simulink model "Base_INS"  (R2018b)
settings: configuration reference "ins_config" (kept outside this file)
undefined symbols (not defined in the file): DiscIntNeverNeededParam, INS_CONST, INS_EXPORT, INS_PARAM
libraries: simulink x95, AP_Math x15, Filter x6, Quaternion x2, Rotation x2
(part 1 of 4)
settings Model: SimulationMode=accelerator  Creator=Jiachi  LastModifiedBy=zouji
settings ConfigSetRef: SourceLocation=Base Workspace

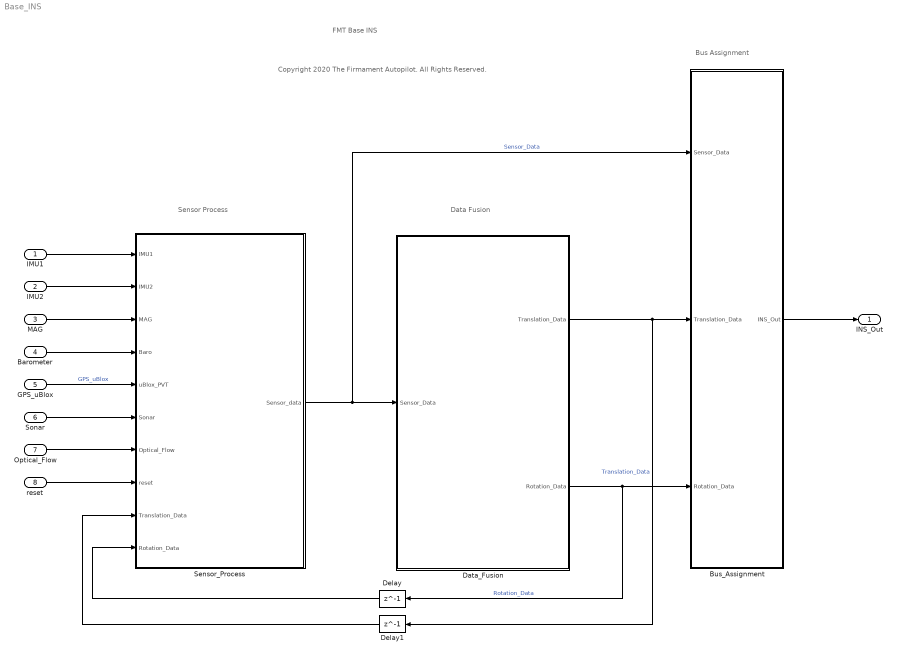
== system Base_INS ==
  note: FMT Base INS
  note: Sensor Process
  note: Data Fusion
  note: Bus Assignment
  note: Copyright 2020 The Firmament Autopilot. All Rights Reserved.
  IMU1 : Inport  OutDataTypeStr=Bus: IMU_Bus  PortDimensions=[1 1]  SampleTime=[INS_CONST.dt,0]  Interpolate=off  BusOutputAsStruct=on
  IMU2 : Inport  Port=2  OutDataTypeStr=Bus: IMU_Bus  PortDimensions=[1 1]  SampleTime=[INS_CONST.dt,0]  Interpolate=off  BusOutputAsStruct=on
  MAG : Inport  Port=3  OutDataTypeStr=Bus: MAG_Bus  PortDimensions=[1 1]  SampleTime=[INS_CONST.dt,0]  Interpolate=off  BusOutputAsStruct=on
  Barometer : Inport  Port=4  OutDataTypeStr=Bus: Barometer_Bus  PortDimensions=[1 1]  SampleTime=[INS_CONST.dt,0]  Interpolate=off  BusOutputAsStruct=on
  GPS_uBlox : Inport  Port=5  OutDataTypeStr=Bus: GPS_uBlox_Bus  PortDimensions=[1 1]  SampleTime=[INS_CONST.dt,0]  Interpolate=off  BusOutputAsStruct=on
  Sonar : Inport  Port=6  OutDataTypeStr=Bus: Sonar_Bus  PortDimensions=1  SampleTime=[INS_CONST.dt,0]  Interpolate=off  BusOutputAsStruct=on
  Optical_Flow : Inport  Port=7  OutDataTypeStr=Bus: Optical_Flow_Bus  PortDimensions=[1 1]  SampleTime=[INS_CONST.dt,0]  Interpolate=off  BusOutputAsStruct=on
  reset : Inport  Port=8  OutDataTypeStr=uint8  PortDimensions=1
  Bus_Assignment : Subsystem  TreatAsAtomicUnit=on
  Data_Fusion : Subsystem  TreatAsAtomicUnit=on
  Delay : Delay  DelayLength=1
  Delay1 : Delay  DelayLength=1
  Sensor_Process : Subsystem  TreatAsAtomicUnit=on
  INS_Out : Outport  OutDataTypeStr=Bus: INS_Out_Bus
  wires:
  IMU1/1 -> Sensor_Process/1(IMU1)
  MAG/1 -> Sensor_Process/3(MAG)
  Barometer/1 -> Sensor_Process/4(Baro)
  GPS_uBlox/1 -> Sensor_Process/5(uBlox_PVT)  "GPS_uBlox"
  Sonar/1 -> Sensor_Process/6(Sonar)
  Bus_Assignment/1(INS_Out) -> INS_Out/1
  reset/1 -> Sensor_Process/8(reset)
  Optical_Flow/1 -> Sensor_Process/7(Optical_Flow)
  IMU2/1 -> Sensor_Process/2(IMU2)
  Sensor_Process/1(Sensor_data) -> Bus_Assignment/1(Sensor_Data), Data_Fusion/1(Sensor_Data)  "Sensor_Data"
  Data_Fusion/2(Rotation_Data) -> Delay/1, Bus_Assignment/3(Rotation_Data)  "Rotation_Data"
  Data_Fusion/1(Translation_Data) -> Delay1/1, Bus_Assignment/2(Translation_Data)  "Translation_Data"
  Delay/1 -> Sensor_Process/10(Rotation_Data)
  Delay1/1 -> Sensor_Process/9(Translation_Data)

== system Base_INS/Bus_Assignment ==
  Sensor_Data : Inport
  Translation_Data : Inport  Port=2
  Rotation_Data : Inport  Port=3
  Bus Creator : BusCreator  Inputs=24  OutDataTypeStr=Bus: INS_Out_Bus
      settings: InheritFromInputs=off
  Counter : Subsystem  TreatAsAtomicUnit=on
  Rotation_Output : Subsystem  TreatAsAtomicUnit=on
  Status_Output : Subsystem  TreatAsAtomicUnit=on
  Translation_Output : Subsystem  TreatAsAtomicUnit=on
  INS_Out : Outport  OutDataTypeStr=Bus: INS_Out_Bus
  wires:
  Bus Creator/1 -> INS_Out/1
  Counter/1(timestamp_ms) -> Bus Creator/1  "timestamp"
  Rotation_Output/2(theta) -> Bus Creator/3  "theta"
  Rotation_Output/1(phi) -> Bus Creator/2  "phi"
  Rotation_Output/4(att_quat) -> Bus Creator/5  "quat"
  Rotation_Output/3(psi) -> Bus Creator/4  "psi"
  Rotation_Output/5(p) -> Bus Creator/6  "p"
  Rotation_Output/6(q) -> Bus Creator/7  "q"
  Rotation_Output/7(r) -> Bus Creator/8  "r"
  Rotation_Output/8(sfor_x) -> Bus Creator/9  "ax"
  Rotation_Output/9(sfor_y) -> Bus Creator/10  "ay"
  Rotation_Output/10(sfor_z) -> Bus Creator/11  "az"
  Translation_Output/1(velN) -> Bus Creator/12  "vn"
  Translation_Output/2(velE) -> Bus Creator/13  "ve"
  Translation_Output/3(velD) -> Bus Creator/14  "vd"
  Translation_Output/5(longitude) -> Bus Creator/16  "lon"
  Translation_Output/6(latitude) -> Bus Creator/17  "lat"
  Translation_Output/7(altitude) -> Bus Creator/18  "alt"
  Status_Output/1(flag) -> Bus Creator/23  "flag"
  Status_Output/2(status) -> Bus Creator/24  "status"
  Translation_Output/8(x_R_m) -> Bus Creator/19  "x_R"
  Translation_Output/9(y_R_m) -> Bus Creator/20  "y_R"
  Translation_Output/10(h_R_m) -> Bus Creator/21  "h_R"
  Translation_Output/11(h_AGL_m) -> Bus Creator/22  "h_AGL"
  Translation_Output/4(reserved) -> Bus Creator/15  "reserved"
  Translation_Data/1 -> Status_Output/1(Translation_Data), Translation_Output/1(Translation_Data), Rotation_Output/2(Translation_Data)
  Rotation_Data/1 -> Status_Output/2(Rotation_Data), Rotation_Output/1(Rotation_Data)
  Sensor_Data/1 -> Status_Output/3(Sensor_Data)

== system Base_INS/Data_Fusion ==
  note: AHRS
  note: Translaton Filter
  Sensor_Data : Inport
  AHRS : Subsystem
  Translation_Filter : Subsystem
  Translation_Data : Outport
  Rotation_Data : Outport  Port=2
  wires:
  AHRS/1(Rotation_Data) -> Rotation_Data/1, Translation_Filter/2(Rotation_Data)
  Translation_Filter/1(Translation_Data) -> Translation_Data/1
  Sensor_Data/1 -> Translation_Filter/1(Sensor_Data), AHRS/1(Sensor_Data)

== system Base_INS/Sensor_Process ==
  IMU1 : Inport  Interpolate=off  BusOutputAsStruct=on
  IMU2 : Inport  Port=2  Interpolate=off  BusOutputAsStruct=on
  MAG : Inport  Port=3  Interpolate=off  BusOutputAsStruct=on
  Baro : Inport  Port=4  Interpolate=off  BusOutputAsStruct=on
  uBlox_PVT : Inport  Port=5  Interpolate=off  BusOutputAsStruct=on
  Sonar : Inport  Port=6  PortDimensions=[1 1]  Interpolate=off  BusOutputAsStruct=on
  Optical_Flow : Inport  Port=7
  reset : Inport  Port=8
  Translation_Data : Inport  Port=9
  Rotation_Data : Inport  Port=10
  Baro_Process : Subsystem  TreatAsAtomicUnit=on
  Bus Creator : BusCreator  Inputs=7
  GPS_Process : Subsystem  TreatAsAtomicUnit=on
  IMU_Process : Subsystem  TreatAsAtomicUnit=on
  Mag_Process : Subsystem  TreatAsAtomicUnit=on
  Optical_Flow_Preprocessing : Subsystem  TreatAsAtomicUnit=on
  Signal Conversion : SignalConversion  OverrideOpt=off
  Sonar_Process : Subsystem  TreatAsAtomicUnit=on
  Sensor_data : Outport
  wires:
  Translation_Data/1 -> Sonar_Process/1(Translation_Data)
  Sonar_Process/1(Sonar_Data) -> Bus Creator/5  "Sonar_Data"
  Sonar/1 -> Sonar_Process/2(Sonar)
  IMU1/1 -> IMU_Process/1(IMU1)
  uBlox_PVT/1 -> GPS_Process/1(uBlox_PVT)
  GPS_Process/1(GPS_Data) -> Mag_Process/3(GPS_Data), Bus Creator/3  "GPS_Data"
  MAG/1 -> Mag_Process/1(Mag)
  Rotation_Data/1 -> Optical_Flow_Preprocessing/1(Rotation_Data), Mag_Process/2(Rotation_Data)
  Baro/1 -> Baro_Process/1(Baro)
  IMU_Process/1(IMU_Data) -> Bus Creator/1  "IMU_Data"
  Mag_Process/1(Mag_Data) -> Bus Creator/2  "Mag_Data"
  reset/1 -> Signal Conversion/1
  Signal Conversion/1 -> Bus Creator/7  "global_reset"
  Baro_Process/1(Baro_Data) -> Bus Creator/4  "Baro_Data"
  Bus Creator/1 -> Sensor_data/1
  Optical_Flow/1 -> Optical_Flow_Preprocessing/2(Vision_Flow)
  Optical_Flow_Preprocessing/1(VisionFlow_Data) -> Bus Creator/6  "VisionFlow_Data"
  IMU2/1 -> IMU_Process/2(IMU2)

== system Base_INS/Bus_Assignment/Counter ==
  Add : Sum
  Constant : Constant  Value=INS_EXPORT.period  OutDataTypeStr=uint32
  Data Type Conversion : DataTypeConversion  OutDataTypeStr=uint32
  Output : UnitDelay  InitialCondition=0.0  SampleTime=-1
  timestamp_ms : Outport
  wires:
  Add/1 -> Output/1
  Output/1 -> Add/2, Data Type Conversion/1
  Data Type Conversion/1 -> timestamp_ms/1
  Constant/1 -> Add/1

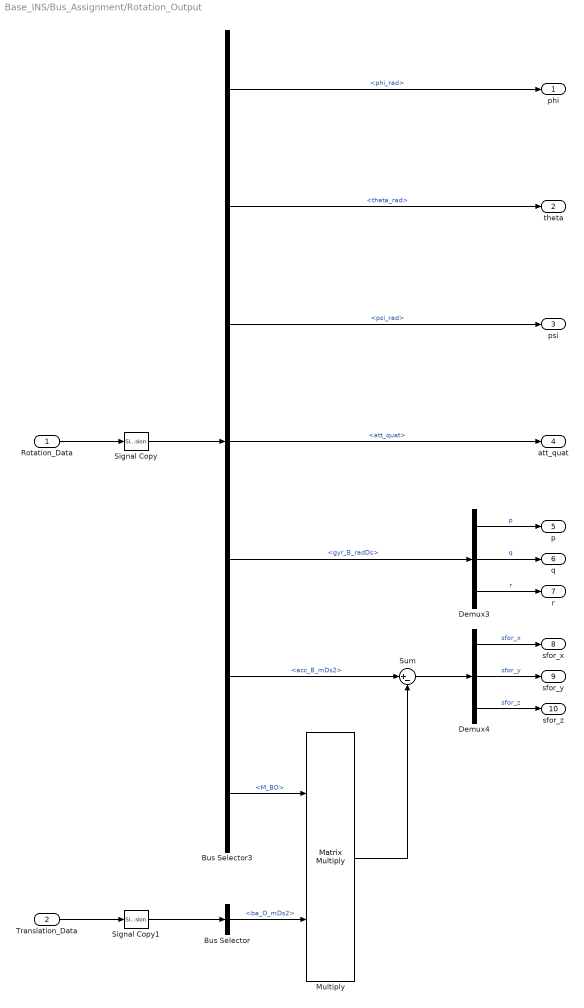
== system Base_INS/Bus_Assignment/Rotation_Output ==
  Rotation_Data : Inport
  Translation_Data : Inport  Port=2
  Bus Selector : BusSelector  OutputSignals=ba_O_mDs2
  Bus Selector3 : BusSelector  OutputSignals=phi_rad,theta_rad,psi_rad,att_quat,gyr_B_radDs,acc_B_mDs2,M_BO
  Demux3 : Demux  Outputs=3
  Demux4 : Demux  Outputs=3
  Multiply : Product  Multiplication=Matrix(*)
  Signal Copy : SignalConversion  OverrideOpt=off
  Signal Copy1 : SignalConversion  OverrideOpt=off
  Sum : Sum  Inputs=|+-
  phi : Outport
  theta : Outport  Port=2
  psi : Outport  Port=3
  att_quat : Outport  Port=4
  p : Outport  Port=5
  q : Outport  Port=6
  r : Outport  Port=7
  sfor_x : Outport  Port=8
  sfor_y : Outport  Port=9
  sfor_z : Outport  Port=10
  wires:
  Bus Selector/1 -> Multiply/2  "<ba_O_mDs2>"
  Demux4/1 -> sfor_x/1  "sfor_x"
  Demux3/3 -> r/1  "r"
  Demux3/2 -> q/1  "q"
  Demux3/1 -> p/1  "p"
  Bus Selector3/5 -> Demux3/1  "<gyr_B_radDs>"
  Sum/1 -> Demux4/1
  Bus Selector3/1 -> phi/1  "<phi_rad>"
  Bus Selector3/6 -> Sum/1  "<acc_B_mDs2>"
  Demux4/3 -> sfor_z/1  "sfor_z"
  Demux4/2 -> sfor_y/1  "sfor_y"
  Bus Selector3/2 -> theta/1  "<theta_rad>"
  Bus Selector3/3 -> psi/1  "<psi_rad>"
  Bus Selector3/7 -> Multiply/1  "<M_BO>"
  Multiply/1 -> Sum/2
  Bus Selector3/4 -> att_quat/1  "<att_quat>"
  Rotation_Data/1 -> Signal Copy/1
  Translation_Data/1 -> Signal Copy1/1
  Signal Copy/1 -> Bus Selector3/1
  Signal Copy1/1 -> Bus Selector/1

== system Base_INS/Bus_Assignment/Status_Output ==
  Translation_Data : Inport
  Rotation_Data : Inport  Port=2
  Sensor_Data : Inport  Port=3
  Bus Selector2 : BusSelector  OutputSignals=standstill
  INS_Flag : Subsystem
  INS_Quality : Subsystem
  INS_Ready : Subsystem
  Sensor_Status : Subsystem
  flag : Outport
  status : Outport  Port=2
  wires:
  INS_Flag/1(flags) -> flag/1
  Sensor_Status/1(status) -> status/1
  INS_Quality/1(Quality) -> INS_Flag/2(INS_Quality)
  Rotation_Data/1 -> INS_Ready/2(Rotation_Data), Bus Selector2/1
  Sensor_Data/1 -> INS_Quality/1(Sensor_Data), INS_Flag/3(Sensor_Data), Sensor_Status/1(Sensor_Data)
  Bus Selector2/1 -> INS_Flag/4(standstill)  "<standstill>"
  Translation_Data/1 -> INS_Ready/1(Translation_Data)
  INS_Ready/1(INS_Ready) -> INS_Flag/1(INS_ready)

== system Base_INS/Bus_Assignment/Translation_Output ==
  Translation_Data : Inport
  Bus Selector4 : BusSelector  OutputSignals=vel_N_mDs,vel_E_mDs,vel_D_mDs,mue_rad,lambda_rad,h_m,x_R_m,y_R_m,h_R_m,h_gnd_m
  Constant : Constant  Value=0  OutDataTypeStr=single
  Signal Copy : SignalConversion  OverrideOpt=off
  velN : Outport
  velE : Outport  Port=2
  velD : Outport  Port=3
  reserved : Outport  Port=4
  longitude : Outport  Port=5
  latitude : Outport  Port=6
  altitude : Outport  Port=7
  x_R_m : Outport  Port=8
  y_R_m : Outport  Port=9
  h_R_m : Outport  Port=10
  h_AGL_m : Outport  Port=11
  wires:
  Translation_Data/1 -> Signal Copy/1
  Bus Selector4/4 -> latitude/1  "<mue_rad>"
  Bus Selector4/5 -> longitude/1  "<lambda_rad>"
  Bus Selector4/2 -> velE/1  "<vel_E_mDs>"
  Bus Selector4/3 -> velD/1  "<vel_D_mDs>"
  Bus Selector4/6 -> altitude/1  "<h_m>"
  Bus Selector4/1 -> velN/1  "<vel_N_mDs>"
  Bus Selector4/10 -> h_AGL_m/1  "<h_gnd_m>"
  Bus Selector4/9 -> h_R_m/1  "<h_R_m>"
  Bus Selector4/7 -> x_R_m/1  "<x_R_m>"
  Bus Selector4/8 -> y_R_m/1  "<y_R_m>"
  Constant/1 -> reserved/1
  Signal Copy/1 -> Bus Selector4/1

== system Base_INS/Data_Fusion/AHRS ==
  Sensor_Data : Inport
  Attitude_Init : Subsystem  TreatAsAtomicUnit=on
  Correct : Subsystem  TreatAsAtomicUnit=on
  Delay : Delay  DelayLength=1
  Integrate : Subsystem  TreatAsAtomicUnit=on
  Rotation_Data : Outport
  wires:
  Correct/1(rot_B_correction) -> Integrate/1(rot_B_correction)
  Correct/2(bias_g_correction) -> Integrate/2(bias_g_correction)
  Attitude_Init/1(standstill) -> Integrate/3(standstill), Correct/3(standstill)
  Integrate/1(Rotation_Data) -> Rotation_Data/1, Delay/1
  Attitude_Init/3(quat_0) -> Integrate/5(quat_0)
  Attitude_Init/2(att_reset) -> Integrate/4(att_reset)
  Sensor_Data/1 -> Integrate/6(Sensor_Data), Correct/2(Sensor_Data), Attitude_Init/1(Sensor_Data)
  Delay/1 -> Correct/1(Rotation_Data)

== system Base_INS/Data_Fusion/Translation_Filter ==
  Sensor_Data : Inport
  Rotation_Data : Inport  Port=2
  CF : Subsystem  TreatAsAtomicUnit=on
  Delay : Delay  DelayLength=1
  Process : Subsystem  TreatAsAtomicUnit=on
  Translation_Data : Outport
  wires:
  CF/1(Translation_Data) -> Delay/1, Translation_Data/1
  Process/1(Processed_Data) -> CF/1(Processed_Data)  "Processed_Data"
  Rotation_Data/1 -> CF/2(Rotation_Data), Process/2(Rotation_Data)
  Sensor_Data/1 -> Process/1(Sensor_Data)
  Delay/1 -> Process/3(Translation_Data)

== system Base_INS/Sensor_Process/Baro_Process ==
  Baro : Inport
  Bus Creator : BusCreator  Inputs=5
  Bus Selector1 : BusSelector  OutputSignals=pressure
  Bus Selector2 : BusSelector  OutputSignals=temperature,timestamp
  P1 : Constant  Value=101.325  OutDataTypeStr=Inherit: Inherit via back propagation
  Pressure_Height : Subsystem
  Relative_Height : Subsystem  mask{pressure_min=30e3, pressure_max=110e3, temp_min=-30, temp_max=80, s_first=500, s_last=1000}
      mask prompts: pressure_min "Min. valid pressure"; pressure_max "Max. valid pressure"; temp_min "Min. valid temperature"; temp_max "Max. valid temperature"; s_first "First Sample for Initial Averaging"; s_last "Last Sample for Initial Averaging"
  Baro_Data : Outport
  wires:
  Bus Selector1/1 -> Pressure_Height/1(p_Pa)  "<pressure>"
  P1/1 -> Pressure_Height/2(QNH_kPa)
  Relative_Height/2(valid) -> Bus Creator/2  "baro_valid"
  Baro/1 -> Bus Selector2/1, Bus Selector1/1, Relative_Height/1(Baro)
  Relative_Height/1(h_R_m) -> Bus Creator/1  "h_R_m"
  Pressure_Height/1(h_FL_m) -> Bus Creator/3  "h_FL_m"
  Bus Creator/1 -> Baro_Data/1
  Bus Selector2/1 -> Bus Creator/4  "<temperature>"
  Bus Selector2/2 -> Bus Creator/5  "<timestamp>"

== system Base_INS/Sensor_Process/GPS_Process ==
  uBlox_PVT : Inport  Interpolate=off  BusOutputAsStruct=on
  Bus Creator1 : BusCreator  Inputs=16
  Compare To Constant : simulink/Logic and Bit Operations/Compare To Constant  relop=>  const=0  OutDataTypeStr=boolean
  Compare To Constant1 : simulink/Logic and Bit Operations/Compare To Constant  relop=<  const=2  OutDataTypeStr=boolean
  GPS_Status_and_Quality : Subsystem
  Scaling : Subsystem
  WGS84_Model : Subsystem
  GPS_Data : Outport
  wires:
  Compare To Constant1/1 -> Bus Creator1/1  "GPS_reset"
  WGS84_Model/5(dz_dh) -> Bus Creator1/8  "dz_dh"
  uBlox_PVT/1 -> Scaling/1(uBlox_PVT), GPS_Status_and_Quality/1(uBlox_PVT)
  Compare To Constant/1 -> WGS84_Model/Trigger
  Bus Creator1/1 -> GPS_Data/1
  GPS_Status_and_Quality/1(gps_status) -> Compare To Constant1/1, Compare To Constant/1  "Status"
  WGS84_Model/2(lat_0_rad) -> Bus Creator1/5  "lat_0_rad"
  WGS84_Model/3(dx_dlat) -> Bus Creator1/6
  WGS84_Model/4(dy_dlon) -> Bus Creator1/7
  GPS_Status_and_Quality/2(speed_quality) -> Bus Creator1/2  "sqd_quality"
  GPS_Status_and_Quality/3(pos_quality) -> Bus Creator1/3  "pos_quality"
  Scaling/2(lon_rad) -> WGS84_Model/2(lon), Bus Creator1/10  "lambda_rad"
  Scaling/3(height_m) -> WGS84_Model/3(height), Bus Creator1/11  "height_m"
  Scaling/1(lat_rad) -> Bus Creator1/9, WGS84_Model/1(lat)  "mue_rad"
  Scaling/4(vel_N) -> Bus Creator1/12  "vn_mPs"
  Scaling/5(vel_E) -> Bus Creator1/13  "ve_mPs"
  Scaling/6(vel_D) -> Bus Creator1/14  "vd_mPs"
  Scaling/7(numSV) -> Bus Creator1/15  "numSV"
  Scaling/8(timestamp_ms) -> Bus Creator1/16  "timestamp_ms"
  WGS84_Model/1(lon_0_rad) -> Bus Creator1/4  "lon_0_rad"

== system Base_INS/Sensor_Process/IMU_Process ==
  IMU1 : Inport
  IMU2 : Inport  Port=2
  Bus Creator : BusCreator  Inputs=4
  Bus_Assignment : Subsystem
  IMU1_Scaling : Subsystem
  IMU1_Valid_Check : Subsystem  mask{gyr_min=-2200*pi/180, gyr_max=2200*pi/180, acc_min=-10*INS_CONST.g, acc_max=10*INS_CONST.g, timeout=100}
      mask prompts: gyr_min "Gyro Min Value"; gyr_max "Gyro Max Value"; acc_min "Accel Min Value"; acc_max "Accel Max Value"; timeout "Timeout in ms"
  IMU2_Scaling : Subsystem
  IMU2_Valid_Check : Subsystem  mask{gyr_min=-2200*pi/180, gyr_max=2200*pi/180, acc_min=-10*INS_CONST.g, acc_max=10*INS_CONST.g, timeout=100}
      mask prompts: gyr_min "Gyro Min Value"; gyr_max "Gyro Max Value"; acc_min "Accel Min Value"; acc_max "Accel Max Value"; timeout "Timeout in ms"
  IMU_Data : Outport
  wires:
  Bus Creator/1 -> IMU_Data/1
  IMU2_Scaling/3(timestamp_ms) -> IMU2_Valid_Check/3(timestamp_ms)
  IMU2_Scaling/2(acc_B_mDs2) -> IMU2_Valid_Check/2(acc_B_mDs2), Bus_Assignment/5(IMU2_acc_B_mPs2)
  IMU2_Scaling/1(gyr_B_radDs) -> IMU2_Valid_Check/1(gyr_B_radDs), Bus_Assignment/4(IMU2_gyr_B_radPs)
  IMU2/1 -> IMU2_Scaling/1(IMU2)
  IMU1_Scaling/1(gyr_B_radDs) -> IMU1_Valid_Check/1(gyr_B_radDs), Bus_Assignment/1(IMU1_gyr_B_radPs)
  IMU1/1 -> IMU1_Scaling/1(IMU1)
  IMU1_Scaling/3(timestamp_ms) -> IMU1_Valid_Check/3(timestamp_ms)
  IMU1_Scaling/2(acc_B_mDs2) -> IMU1_Valid_Check/2(acc_B_mDs2), Bus_Assignment/2(IMU1_acc_B_mPs2)
  IMU1_Valid_Check/1(valid) -> Bus_Assignment/3(IMU1_valid)  "IMU1_valid"
  IMU2_Valid_Check/1(valid) -> Bus_Assignment/6(IMU2_valid)  "IMU2_valid"
  Bus_Assignment/1(gyr_B_radPs) -> Bus Creator/1  "gyr_B_radPs"
  Bus_Assignment/2(acc_B_mPs2) -> Bus Creator/2  "acc_B_mPs2"
  Bus_Assignment/3(IMU_status) -> Bus Creator/3  "IMU_status"
  Bus_Assignment/4(IMU_valid) -> Bus Creator/4  "IMU_valid"

== system Base_INS/Sensor_Process/Mag_Process ==
  Mag : Inport
  Rotation_Data : Inport  Port=2
  GPS_Data : Inport  Port=3
  Bus Creator : BusCreator  Inputs=2
  Bus Selector : BusSelector  OutputSignals=timestamp
  Bus Selector2 : BusSelector  OutputSignals=mag_x,mag_y,mag_z
  Bus Selector4 : BusSelector  OutputSignals=M_OB
  Mag_Scaling : Subsystem
  Mag_Valid_Check : Subsystem  mask{mag_min=-30000, mag_max=30000, timeout=1000}
      mask prompts: mag_min "Min Mag Value"; mag_max "Max Mag Value"; timeout "Timeout in ms"
  Magnetometer : Subsystem
  Vector Concatenate2 : Concatenate  NumInputs=3  Mode=Multidimensional array
  Mag_Data : Outport
  wires:
  Rotation_Data/1 -> Bus Selector4/1
  Vector Concatenate2/1 -> Mag_Valid_Check/1(mag_B_gauss), Mag_Scaling/1(mag_B_gauss)
  Bus Selector2/2 -> Vector Concatenate2/2  "<mag_y>"
  Bus Selector2/1 -> Vector Concatenate2/1  "<mag_x>"
  Bus Selector4/1 -> Magnetometer/3(M_OB)  "<M_OB>"
  Mag_Valid_Check/1(valid) -> Magnetometer/2(Mag_valid)
  Bus Selector2/3 -> Vector Concatenate2/3  "<mag_z>"
  Mag_Scaling/1(mag_B_uT) -> Magnetometer/1(mag_B_uT)
  Mag/1 -> Bus Selector/1, Bus Selector2/1
  Magnetometer/1(mag_normalized_B) -> Bus Creator/1  "mag_norm_B"
  GPS_Data/1 -> Magnetometer/4(GPS_Data)
  Magnetometer/2(mag_Quality) -> Bus Creator/2  "mag_quality"
  Bus Creator/1 -> Mag_Data/1
  Bus Selector/1 -> Mag_Valid_Check/2(timestamp_ms)  "<timestamp>"

== system Base_INS/Sensor_Process/Optical_Flow_Preprocessing ==
  Rotation_Data : Inport
  Vision_Flow : Inport  Port=2
  Bus Creator : BusCreator  Inputs=6
  Bus Selector : BusSelector  OutputSignals=timestamp_ms,valid,vel_x_mPs,vel_y_mPs
  Bus Selector1 : BusSelector  OutputSignals=M_CO
  Constant : Constant  Value=0  OutDataTypeStr=single
  Demux : Demux  Outputs=3
  Multiply : Product  Multiplication=Matrix(*)
  Mux : Mux  Inputs=3
  Signal Copy{,1..3} (4 alike) : SignalConversion  OverrideOpt=off
  Terminator : Terminator
  Valid_Detect : Subsystem
  VisionFlow_Data : Outport
  wires:
  Bus Creator/1 -> VisionFlow_Data/1
  Vision_Flow/1 -> Bus Selector/1
  Bus Selector/3 -> Signal Copy/1, Mux/1  "<vel_x_mPs>"
  Bus Selector/4 -> Signal Copy1/1, Mux/2  "<vel_y_mPs>"
  Signal Copy/1 -> Bus Creator/3  "vel_x_B_mDs"
  Signal Copy1/1 -> Bus Creator/4  "vel_y_B_mDs"
  Bus Selector/1 -> Bus Creator/1, Valid_Detect/1(timestamp_ms)  "<timestamp_ms>"
  Bus Selector/2 -> Valid_Detect/2(vf_valid)  "<valid>"
  Valid_Detect/1(valid) -> Bus Creator/2  "valid"
  Rotation_Data/1 -> Bus Selector1/1
  Signal Copy2/1 -> Bus Creator/5  "vel_x_O_mDs"
  Signal Copy3/1 -> Bus Creator/6  "vel_y_O_mDs"
  Bus Selector1/1 -> Multiply/1  "<M_CO>"
  Constant/1 -> Mux/3
  Mux/1 -> Multiply/2
  Multiply/1 -> Demux/1
  Demux/1 -> Signal Copy2/1
  Demux/2 -> Signal Copy3/1
  Demux/3 -> Terminator/1

== system Base_INS/Sensor_Process/Sonar_Process ==
  Translation_Data : Inport
  Sonar : Inport  Port=2
  Bus Creator : BusCreator  Inputs=3
  Bus Selector : BusSelector  OutputSignals=timestamp_ms,distance_m
  Signal Conversion : SignalConversion  OverrideOpt=off
  Signal Conversion1 : SignalConversion  OverrideOpt=off
  Valid_Check : Subsystem
  Sonar_Data : Outport
  wires:
  Translation_Data/1 -> Valid_Check/3(Translation_Data)
  Bus Creator/1 -> Sonar_Data/1
  Signal Conversion/1 -> Bus Creator/2  "distance_m"
  Sonar/1 -> Bus Selector/1
  Bus Selector/2 -> Valid_Check/2(diatance_m), Signal Conversion/1  "<distance_m>"
  Bus Selector/1 -> Signal Conversion1/1, Valid_Check/1(timestamp_ms)  "<timestamp_ms>"
  Valid_Check/1(sonar_valid) -> Bus Creator/3  "sonar_valid"
  Signal Conversion1/1 -> Bus Creator/1  "timestamp_ms"

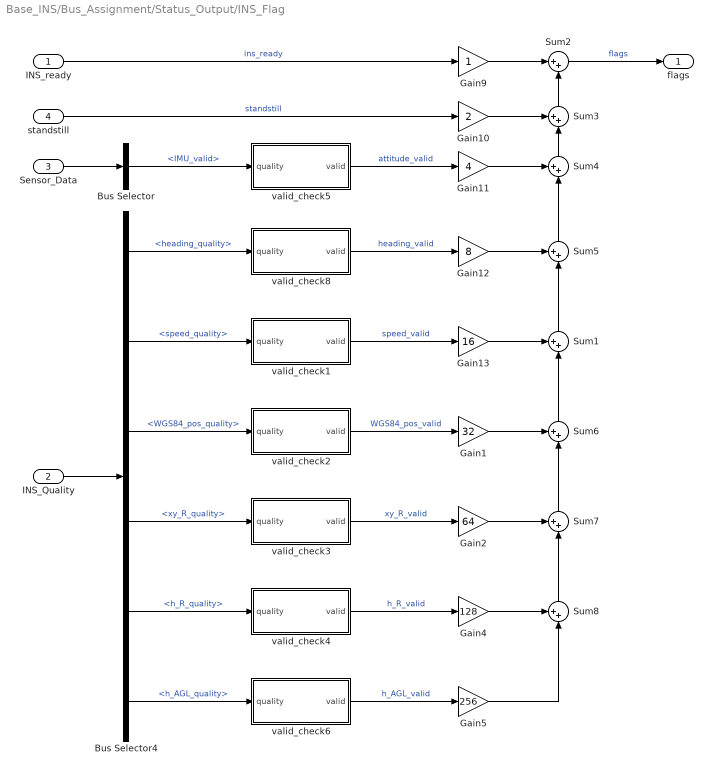
== system Base_INS/Bus_Assignment/Status_Output/INS_Flag ==
  INS_ready : Inport
  INS_Quality : Inport  Port=2
  Sensor_Data : Inport  Port=3
  standstill : Inport  Port=4
  Bus Selector : BusSelector  OutputSignals=IMU_Data.IMU_valid
  Bus Selector4 : BusSelector  OutputSignals=heading_quality,speed_quality,WGS84_pos_quality,xy_R_quality,h_R_quality,h_AGL_quality
  Gain1 : Gain  Gain=32  OutDataTypeStr=uint32
  Gain10 : Gain  Gain=2  OutDataTypeStr=uint32
  Gain11 : Gain  Gain=4  OutDataTypeStr=uint32
  Gain12 : Gain  Gain=8  OutDataTypeStr=uint32
  Gain13 : Gain  Gain=16  OutDataTypeStr=uint32
  Gain2 : Gain  Gain=64  OutDataTypeStr=uint32
  Gain4 : Gain  Gain=128  OutDataTypeStr=uint32
  Gain5 : Gain  Gain=256  OutDataTypeStr=uint32
  Gain9 : Gain  OutDataTypeStr=uint32
  Sum{1,3..8} (7 alike) : Sum  Inputs=++|
  Sum2 : Sum  Inputs=|++
  valid_check1 : Subsystem  mask{time_out=1000}
      mask prompts: time_out "timeout in ms"
  valid_check2 : Subsystem  mask{time_out=1000}
      mask prompts: time_out "timeout in ms"
  valid_check3 : Subsystem  mask{time_out=1000}
      mask prompts: time_out "timeout in ms"
  valid_check4 : Subsystem  mask{time_out=200}
      mask prompts: time_out "timeout in ms"
  valid_check5 : Subsystem  mask{time_out=100}
      mask prompts: time_out "timeout in ms"
  valid_check6 : Subsystem  mask{time_out=100}
      mask prompts: time_out "timeout in ms"
  valid_check8 : Subsystem  mask{time_out=1000}
      mask prompts: time_out "timeout in ms"
  flags : Outport
  wires:
  INS_ready/1 -> Gain9/1  "ins_ready"
  Bus Selector/1 -> valid_check5/1(quality)  "<IMU_valid>"
  Gain1/1 -> Sum6/1
  Sum1/1 -> Sum5/2
  Gain13/1 -> Sum1/1
  valid_check2/1(valid) -> Gain1/1  "WGS84_pos_valid"
  valid_check1/1(valid) -> Gain13/1  "speed_valid"
  valid_check5/1(valid) -> Gain11/1  "attitude_valid"
  Bus Selector4/3 -> valid_check2/1(quality)  "<WGS84_pos_quality>"
  Bus Selector4/2 -> valid_check1/1(quality)  "<speed_quality>"
  Bus Selector4/1 -> valid_check8/1(quality)  "<heading_quality>"
  INS_Quality/1 -> Bus Selector4/1
  Sum2/1 -> flags/1  "flags"
  Sum5/1 -> Sum4/2
  Gain9/1 -> Sum2/1
  Gain11/1 -> Sum4/1
  Gain12/1 -> Sum5/1
  Sum3/1 -> Sum2/2
  Sum4/1 -> Sum3/2
  Sensor_Data/1 -> Bus Selector/1
  Gain10/1 -> Sum3/1
  Sum6/1 -> Sum1/2
  Sum7/1 -> Sum6/2
  standstill/1 -> Gain10/1  "standstill"
  valid_check3/1(valid) -> Gain2/1  "xy_R_valid"
  valid_check4/1(valid) -> Gain4/1  "h_R_valid"
  Gain2/1 -> Sum7/1
  Sum8/1 -> Sum7/2
  Gain4/1 -> Sum8/1
  Gain5/1 -> Sum8/2
  valid_check6/1(valid) -> Gain5/1  "h_AGL_valid"
  Bus Selector4/4 -> valid_check3/1(quality)  "<xy_R_quality>"
  Bus Selector4/5 -> valid_check4/1(quality)  "<h_R_quality>"
  Bus Selector4/6 -> valid_check6/1(quality)  "<h_AGL_quality>"
  valid_check8/1(valid) -> Gain12/1  "heading_valid"

== system Base_INS/Bus_Assignment/Status_Output/INS_Quality ==
  Sensor_Data : Inport
  Bus Creator : BusCreator  Inputs=6
  Bus Selector : BusSelector  OutputSignals=GPS_Data.sqd_quality
  Bus Selector1 : BusSelector  OutputSignals=GPS_Data.pos_quality
  Bus Selector2 : BusSelector  OutputSignals=Mag_Data.mag_quality
  Bus Selector3 : BusSelector  OutputSignals=GPS_Data.sqd_quality
  Bus Selector4 : BusSelector  OutputSignals=VisionFlow_Data.valid
  Bus Selector5 : BusSelector  OutputSignals=Baro_Data.baro_valid
  Bus Selector6 : BusSelector  OutputSignals=Sonar_Data.sonar_valid
  Data Type Conversion : DataTypeConversion  OutDataTypeStr=single
  Data Type Conversion1 : DataTypeConversion  OutDataTypeStr=single
  Data Type Conversion2 : DataTypeConversion  OutDataTypeStr=single
  Max : MinMax  Function=max  Inputs=2
  Max1 : MinMax  Function=max  Inputs=2
  Max2 : MinMax  Function=max  Inputs=3
  Signal Copy : SignalConversion  OverrideOpt=off
  Signal Copy1 : SignalConversion  OverrideOpt=off
  Signal Copy2 : SignalConversion  OverrideOpt=off
  Quality : Outport
  wires:
  Bus Creator/1 -> Quality/1
  Max/1 -> Bus Creator/3  "heading_quality"
  Sensor_Data/1 -> Bus Selector/1, Bus Selector1/1, Bus Selector6/1, Bus Selector5/1, Bus Selector4/1, Bus Selector2/1, Bus Selector3/1
  Bus Selector2/1 -> Max/2  "<mag_quality>"
  Bus Selector3/1 -> Max/1  "<sqd_quality>"
  Bus Selector/1 -> Signal Copy1/1  "<sqd_quality>"
  Bus Selector1/1 -> Max2/1, Max1/1, Signal Copy/1  "<pos_quality>"
  Signal Copy/1 -> Bus Creator/2  "WGS84_pos_quality"
  Signal Copy1/1 -> Bus Creator/1  "speed_quality"
  Bus Selector4/1 -> Data Type Conversion/1  "<valid>"
  Max1/1 -> Bus Creator/4  "xy_R_quality"
  Bus Selector5/1 -> Data Type Conversion1/1  "<baro_valid>"
  Bus Selector6/1 -> Data Type Conversion2/1  "<sonar_valid>"
  Max2/1 -> Bus Creator/5  "h_R_quality"
  Signal Copy2/1 -> Bus Creator/6  "h_AGL_quality"
  Data Type Conversion/1 -> Max1/2
  Data Type Conversion1/1 -> Max2/2
  Data Type Conversion2/1 -> Max2/3, Signal Copy2/1

== system Base_INS/Bus_Assignment/Status_Output/INS_Ready ==
  Translation_Data : Inport
  Rotation_Data : Inport  Port=2
  Bus Selector1 : BusSelector  OutputSignals=init_done
  Bus Selector3 : BusSelector  OutputSignals=init_done
  Logical Operator : Logic  AllPortsSameDT=off  OutDataTypeStr=boolean
  INS_Ready : Outport
  wires:
  Translation_Data/1 -> Bus Selector1/1
  Bus Selector1/1 -> Logical Operator/1  "<init_done>"
  Bus Selector3/1 -> Logical Operator/2  "<init_done>"
  Logical Operator/1 -> INS_Ready/1
  Rotation_Data/1 -> Bus Selector3/1

== system Base_INS/Bus_Assignment/Status_Output/Sensor_Status ==
  Sensor_Data : Inport
  Bus Selector : BusSelector  OutputSignals=IMU_Data.IMU_status,Mag_Data.mag_quality,Baro_Data.baro_valid
  Bus Selector1 : BusSelector  OutputSignals=GPS_Data.sqd_quality,GPS_Data.pos_quality
  Bus Selector3 : BusSelector  OutputSignals=Sonar_Data.sonar_valid,VisionFlow_Data.valid
  Compare To Zero : simulink/Logic and Bit Operations/Compare To Zero  relop=>  OutDataTypeStr=boolean
  Compare To Zero1 : simulink/Logic and Bit Operations/Compare To Zero  relop=>  OutDataTypeStr=boolean
  Data Type Conversion : DataTypeConversion
  Gain2 : Gain  Gain=4  OutDataTypeStr=uint32
  Gain3 : Gain  Gain=8  OutDataTypeStr=uint32
  Gain4 : Gain  Gain=16  OutDataTypeStr=uint32
  Gain5 : Gain  Gain=32  OutDataTypeStr=uint32
  Gain7 : Gain  Gain=64  OutDataTypeStr=uint32
  Max : MinMax  Function=max  Inputs=2
  Sum : Sum  Inputs=|++
  Sum{2..5} (4 alike) : Sum  Inputs=++|
  status : Outport
  wires:
  Gain7/1 -> Sum5/2  "optical_flow_available"
  Bus Selector3/1 -> Gain5/1  "<sonar_valid>"
  Max/1 -> Compare To Zero1/1
  Compare To Zero1/1 -> Gain4/1
  Bus Selector1/2 -> Max/2  "<pos_quality>"
  Bus Selector1/1 -> Max/1  "<sqd_quality>"
  Gain5/1 -> Sum5/1  "sonar_available"
  Sum5/1 -> Sum4/2
  Gain4/1 -> Sum4/1  "GPS_available"
  Sum4/1 -> Sum3/2
  Gain3/1 -> Sum3/1  "baro_available"
  Sum3/1 -> Sum2/2
  Gain2/1 -> Sum2/1  "mag_available"
  Compare To Zero/1 -> Gain2/1
  Sum2/1 -> Sum/2
  Bus Selector/3 -> Gain3/1  "<baro_valid>"
  Bus Selector/2 -> Compare To Zero/1  "<mag_quality>"
  Sensor_Data/1 -> Bus Selector/1, Bus Selector3/1, Bus Selector1/1
  Sum/1 -> status/1
  Data Type Conversion/1 -> Sum/1  "IMU1_2_available"
  Bus Selector3/2 -> Gain7/1  "<valid>"
  Bus Selector/1 -> Data Type Conversion/1  "<IMU_status>"

== system Base_INS/Data_Fusion/AHRS/Attitude_Init ==
  Sensor_Data : Inport
  Attitude_Init : Subsystem
  Bus Selector : BusSelector  OutputSignals=IMU_Data.IMU_valid,Mag_Data.mag_quality,global_reset
  Bus Selector1 : BusSelector  OutputSignals=IMU_Data.acc_B_mPs2,Mag_Data.mag_norm_B
  Bus Selector2 : BusSelector  OutputSignals=IMU_Data
  Compare To Constant : simulink/Logic and Bit Operations/Compare To Constant  relop=>=  const=0.2  OutDataTypeStr=boolean
  Onground_Check : Subsystem
  Reset_Condition : Subsystem
  standstill : Outport
  att_reset : Outport  Port=2
  quat_0 : Outport  Port=3
  wires:
  Bus Selector2/1 -> Onground_Check/1(IMU_Data)  "<IMU_Data>"
  Bus Selector1/2 -> Attitude_Init/2(mag_B), Reset_Condition/5(mag_norm_B)  "<mag_norm_B>"
  Sensor_Data/1 -> Bus Selector/1, Bus Selector2/1, Bus Selector1/1
  Onground_Check/1(standstill) -> standstill/1
  Reset_Condition/1(att_reset) -> Attitude_Init/Enable, att_reset/1
  Bus Selector/1 -> Reset_Condition/1(IMU_valid)  "<IMU_valid>"
  Bus Selector/3 -> Reset_Condition/3(global_reset)  "<global_reset>"
  Bus Selector/2 -> Compare To Constant/1  "<mag_quality>"
  Bus Selector1/1 -> Attitude_Init/1(acc_B), Reset_Condition/4(acc_B_mPs2)  "<acc_B_mPs2>"
  Attitude_Init/1(quaternion_0) -> quat_0/1
  Compare To Constant/1 -> Reset_Condition/2(Mag_valid)

== system Base_INS/Data_Fusion/AHRS/Correct ==
  Rotation_Data : Inport
  Sensor_Data : Inport  Port=2
  standstill : Inport  Port=3
  Att_Correction : Subsystem
  Bias_Correction : Subsystem
  Bus Selector1 : BusSelector  OutputSignals=IMU_Data
  rot_B_correction : Outport
  bias_g_correction : Outport  Port=2
  wires:
  Bias_Correction/1(bias_g_correction) -> bias_g_correction/1
  Bus Selector1/1 -> Bias_Correction/4(IMU_Data)  "<IMU_Data>"
  standstill/1 -> Att_Correction/3(standstill), Bias_Correction/3(standstill)
  Att_Correction/1(rot_B_correction) -> rot_B_correction/1, Bias_Correction/1(rot_B_correction)
  Sensor_Data/1 -> Bus Selector1/1, Att_Correction/1(Sensor_Data)
  Rotation_Data/1 -> Bias_Correction/2(Rotation_Data), Att_Correction/2(Rotation_Data)

== system Base_INS/Data_Fusion/AHRS/Integrate ==
  rot_B_correction : Inport
  bias_g_correction : Inport  Port=2
  standstill : Inport  Port=3
  att_reset : Inport  Port=4
  quat_0 : Inport  Port=5
  Sensor_Data : Inport  Port=6
  Att_Init_Done : Subsystem
  Attitude_Integration : Subsystem
  Bias_Integration : Subsystem
  Bus Creator : BusCreator  Inputs=13
  Bus Selector : BusSelector  OutputSignals=IMU_Data.gyr_B_radPs
  Bus Selector1 : BusSelector  OutputSignals=IMU_Data.acc_B_mPs2
  Euler_Angle : Subsystem
  Signal Conversion : SignalConversion  OverrideOpt=off
  Signal Conversion1 : SignalConversion  OverrideOpt=off
  Sum2 : Sum  Inputs=|++
  Rotation_Data : Outport
  wires:
  att_reset/1 -> Attitude_Integration/1(att_reset), Att_Init_Done/1(att_reset), Bus Creator/2  "att_reset"
  Signal Conversion/1 -> Bus Creator/12  "acc_B_mDs2"
  Euler_Angle/1(phi_rad) -> Bus Creator/3  "phi_rad"
  Euler_Angle/2(theta_rad) -> Bus Creator/4  "theta_rad"
  Euler_Angle/3(psi_rad) -> Bus Creator/5  "psi_rad"
  Sensor_Data/1 -> Bus Selector/1, Bus Selector1/1
  standstill/1 -> Signal Conversion1/1
  Bus Selector1/1 -> Signal Conversion/1  "<acc_B_mPs2>"
  Bus Creator/1 -> Rotation_Data/1
  Bias_Integration/2(bias_g) -> Bus Creator/11  "bias_g"
  Attitude_Integration/3(M_BO) -> Euler_Angle/2(M_BO), Bus Creator/9  "M_BO"
  Attitude_Integration/2(M_OB) -> Bus Creator/8  "M_OB"
  Attitude_Integration/1(att_quat) -> Bus Creator/7, Euler_Angle/1(att_quat)  "att_quat"
  Bias_Integration/1(rot_B_cal_radDs) -> Sum2/2, Bus Creator/10  "gyr_B_radDs"
  rot_B_correction/1 -> Sum2/1
  Sum2/1 -> Attitude_Integration/3(rot_IB_B)
  Bus Selector/1 -> Bias_Integration/2(rot_IB_B)  "<gyr_B_radPs>"
  bias_g_correction/1 -> Bias_Integration/1(bias_g_correction)
  quat_0/1 -> Attitude_Integration/2(quat_0)
  Att_Init_Done/1(att_init_done) -> Bus Creator/1  "init_done"
  Euler_Angle/4(M_CO) -> Bus Creator/6  "M_CO"
  Signal Conversion1/1 -> Bus Creator/13  "standstill"

== system Base_INS/Data_Fusion/Translation_Filter/CF ==
  Processed_Data : Inport
  Rotation_Data : Inport  Port=2
  Bus_Assignment : Subsystem
  Constant : Constant  Value=0  OutDataTypeStr=Inherit: Inherit via back propagation
  Horizontal_Filter : Subsystem
  Verticle_Filter : Subsystem
  Translation_Data : Outport
  wires:
  Bus_Assignment/1(Translation_Data) -> Translation_Data/1
  Verticle_Filter/1(States) -> Bus_Assignment/3(Verticle_States)
  Horizontal_Filter/1(States) -> Bus_Assignment/2(Horizontal_States)
  Rotation_Data/1 -> Horizontal_Filter/2(Rotation_Data), Verticle_Filter/2(Rotation_Data)
  Processed_Data/1 -> Bus_Assignment/1(Processed_Data), Verticle_Filter/1(Processed_Data), Horizontal_Filter/1(Processed_Data)
  Constant/1 -> Bus_Assignment/4(sonar_bias)

== system Base_INS/Data_Fusion/Translation_Filter/Process ==
  Sensor_Data : Inport
  Rotation_Data : Inport  Port=2
  Translation_Data : Inport  Port=3
  Process_Data : Subsystem
  Sensor_Meas : Subsystem
  Sensor_Status : Subsystem
  Processed_Data : Outport
  wires:
  Process_Data/1(Proecssed_Data) -> Processed_Data/1
  Rotation_Data/1 -> Sensor_Meas/2(Rotation_Data), Process_Data/3(Rotation_Data)
  Sensor_Meas/1(Sensor_Meas) -> Process_Data/2(Sensor_Meas)
  Sensor_Status/1(Sensor_Status) -> Process_Data/1(Sensor_Status)
  Sensor_Data/1 -> Sensor_Meas/1(Sensor_Data), Sensor_Status/1(Sensor_Data)
  Translation_Data/1 -> Process_Data/4(Translation_Data)

== system Base_INS/Sensor_Process/Baro_Process/Pressure_Height ==
  p_Pa : Inport
  QNH_kPa : Inport  Port=2
  Constant : Constant  OutDataTypeStr=single
  Constant1 : Constant  Value=0.190284  OutDataTypeStr=single
  Constant2 : Constant  OutDataTypeStr=single
  Divide : Product  Inputs=*/
  Gain : Gain  Gain=44307.694
  Gain1 : Gain  Gain=0.001
  Interval Test1 : simulink/Logic and Bit Operations/Interval Test  IntervalClosedRight=off  uplimit=110e3  IntervalClosedLeft=off  lowlimit=30e3  OutDataTypeStr=boolean
  Math Function : Math  Operator=pow  SaturateOnIntegerOverflow=on
  MinMax : MinMax  Function=max  Inputs=2
  Multiply : Product  OutDataTypeStr=single
  Sum : Sum  Inputs=|+-
  h_FL_m : Outport
  wires:
  p_Pa/1 -> Interval Test1/1, Gain1/1
  QNH_kPa/1 -> MinMax/1
  MinMax/1 -> Divide/2
  Constant/1 -> MinMax/2
  Divide/1 -> Math Function/1
  Constant1/1 -> Math Function/2
  Constant2/1 -> Sum/1
  Math Function/1 -> Sum/2
  Sum/1 -> Gain/1
  Gain1/1 -> Divide/1  "p_kPa"
  Interval Test1/1 -> Multiply/1
  Gain/1 -> Multiply/2
  Multiply/1 -> h_FL_m/1

== system Base_INS/Sensor_Process/Baro_Process/Relative_Height ==
  Baro : Inport  Interpolate=off  BusOutputAsStruct=on
  Bus Selector : BusSelector  OutputSignals=pressure,temperature,timestamp
  Init_Status : Subsystem
  Logical Operator1 : Logic  Operator=OR  AllPortsSameDT=off  OutDataTypeStr=boolean
  Logical Operator2 : Logic  Operator=NOT  AllPortsSameDT=off  OutDataTypeStr=boolean
  Product1 : Product  Inputs=**
  Reference_and_Derivative : Subsystem
  Sum2 : Sum  Inputs=|+-
  Switch : Switch  Criteria=u2 ~= 0
  h_R_m : Outport
  valid : Outport  Port=2
  wires:
  Logical Operator2/1 -> Logical Operator1/2
  Logical Operator1/1 -> Switch/2
  Init_Status/2(valid) -> Logical Operator2/1, valid/1
  Bus Selector/3 -> Init_Status/3(timestamp)  "<timestamp>"
  Bus Selector/2 -> Init_Status/2(temp_deg), Reference_and_Derivative/2(temprature_deg)  "<temperature>"
  Bus Selector/1 -> Init_Status/1(p_Pa), Reference_and_Derivative/1(p_Pa), Switch/1, Sum2/1  "<pressure>"
  Baro/1 -> Bus Selector/1
  Init_Status/1(initializing) -> Logical Operator1/1, Reference_and_Derivative/Enable
  Reference_and_Derivative/2(dh_dp) -> Product1/2
  Reference_and_Derivative/1(pressure_R) -> Switch/3
  Switch/1 -> Sum2/2
  Sum2/1 -> Product1/1
  Product1/1 -> h_R_m/1

== system Base_INS/Sensor_Process/GPS_Process/GPS_Status_and_Quality ==
  uBlox_PVT : Inport
  Bus Selector3 : BusSelector  OutputSignals=timestamp,hAcc,sAcc,fixType,vAcc
  Compare To Constant2 : simulink/Logic and Bit Operations/Compare To Constant  relop=>  const=1  OutDataTypeStr=boolean
  Compare To Constant4 : simulink/Logic and Bit Operations/Compare To Constant  relop=<  const=1000  OutDataTypeStr=boolean
  Double : Product  Inputs=3  OutDataTypeStr=single  RndMeth=Zero
  Double1 : Product  Inputs=3  OutDataTypeStr=single  RndMeth=Zero
  GPS_Status : Subsystem
  Saturation : Saturate  UpperLimit=1  LowerLimit=0
  Saturation1 : Saturate  UpperLimit=1  LowerLimit=0
  Terminator : Terminator
  horizontal_acc : Subsystem
  speed_acc : Subsystem
  timestamp_check : Subsystem
  gps_status : Outport
  speed_quality : Outport  Port=2
  pos_quality : Outport  Port=3
  wires:
  Bus Selector3/4 -> GPS_Status/3(fixtype)  "<fixType>"
  uBlox_PVT/1 -> Bus Selector3/1
  Saturation/1 -> Double/2
  Compare To Constant2/1 -> Double/3, Double1/3
  Double/1 -> speed_quality/1
  GPS_Status/1(Status) -> Compare To Constant2/1, gps_status/1
  Bus Selector3/2 -> horizontal_acc/1(hAcc), GPS_Status/2(hAcc)  "<hAcc>"
  Saturation1/1 -> Double1/2
  Double1/1 -> pos_quality/1
  Compare To Constant4/1 -> Double/1, Double1/1
  timestamp_check/1(timeout) -> Compare To Constant4/1, GPS_Status/1(timeout)
  Bus Selector3/1 -> timestamp_check/1(timestamp)  "<timestamp>"
  Bus Selector3/3 -> speed_acc/1(sAcc)  "<sAcc>"
  speed_acc/1(quality) -> Saturation/1
  horizontal_acc/1(quality) -> Saturation1/1
  Bus Selector3/5 -> Terminator/1  "<vAcc>"

== system Base_INS/Sensor_Process/GPS_Process/Scaling ==
  uBlox_PVT : Inport
  Bus Selector2 : BusSelector  OutputSignals=lat,lon,height,velN,velE,velD,numSV,timestamp
  Gain : Gain  Gain=1e-3  OutDataTypeStr=single
  Gain1 : Gain  Gain=1e-3  OutDataTypeStr=single
  Gain2 : Gain  Gain=1e-3  OutDataTypeStr=single
  Scalefactor1 : Gain  Gain=1e-7*pi/180  OutDataTypeStr=double
  Scalefactor2 : Gain  Gain=1e-7*pi/180  OutDataTypeStr=double
  Scalefactor3 : Gain  Gain=1e-3  OutDataTypeStr=double
  lat_rad : Outport
  lon_rad : Outport  Port=2
  height_m : Outport  Port=3
  vel_N : Outport  Port=4
  vel_E : Outport  Port=5
  vel_D : Outport  Port=6
  numSV : Outport  Port=7
  timestamp_ms : Outport  Port=8
  wires:
  Bus Selector2/1 -> Scalefactor1/1  "<lat>"
  Bus Selector2/6 -> Gain2/1  "<velD>"
  Bus Selector2/5 -> Gain1/1  "<velE>"
  Bus Selector2/2 -> Scalefactor2/1  "<lon>"
  Scalefactor1/1 -> lat_rad/1
  Bus Selector2/4 -> Gain/1  "<velN>"
  Bus Selector2/3 -> Scalefactor3/1  "<height>"
  uBlox_PVT/1 -> Bus Selector2/1
  Scalefactor3/1 -> height_m/1
  Scalefactor2/1 -> lon_rad/1
  Gain/1 -> vel_N/1  "vel_N"
  Gain2/1 -> vel_D/1  "vel_D"
  Bus Selector2/8 -> timestamp_ms/1  "<timestamp>"
  Gain1/1 -> vel_E/1  "vel_E"
  Bus Selector2/7 -> numSV/1  "<numSV>"

== system Base_INS/Sensor_Process/GPS_Process/WGS84_Model ==
  lat : Inport
  lon : Inport  Port=2
  height : Inport  Port=3
  Trigger : TriggerPort  VariantControl=Variant  PortDimensions=1
  Scalefactor : Gain  OutDataTypeStr=double
  Scalefactor1 : Gain  OutDataTypeStr=double
  WGS84_Derivatives : Subsystem
  lon_0_rad : Outport  InitialOutput=0
  lat_0_rad : Outport  Port=2  InitialOutput=0
  dx_dlat : Outport  Port=3  InitialOutput=1
  dy_dlon : Outport  Port=4  InitialOutput=1
  dz_dh : Outport  Port=5  InitialOutput=1
  wires:
  WGS84_Derivatives/3(dz_dh) -> dz_dh/1
  height/1 -> WGS84_Derivatives/2(h_0)
  lon/1 -> Scalefactor/1
  lat/1 -> Scalefactor1/1
  WGS84_Derivatives/2(dy_dlon) -> dy_dlon/1
  WGS84_Derivatives/1(dx_dlat) -> dx_dlat/1
  Scalefactor/1 -> lon_0_rad/1
  Scalefactor1/1 -> lat_0_rad/1, WGS84_Derivatives/1(lat_0)

== system Base_INS/Sensor_Process/IMU_Process/Bus_Assignment ==
  IMU1_gyr_B_radPs : Inport
  IMU1_acc_B_mPs2 : Inport  Port=2
  IMU1_valid : Inport  Port=3
  IMU2_gyr_B_radPs : Inport  Port=4
  IMU2_acc_B_mPs2 : Inport  Port=5
  IMU2_valid : Inport  Port=6
  Compare To Zero : simulink/Logic and Bit Operations/Compare To Zero  relop=>  OutDataTypeStr=boolean
  IMU_Select : Subsystem
  IMU_Status : Subsystem
  gyr_B_radPs : Outport
  acc_B_mPs2 : Outport  Port=2
  IMU_status : Outport  Port=3
  IMU_valid : Outport  Port=4
  wires:
  Compare To Zero/1 -> IMU_valid/1
  IMU1_valid/1 -> IMU_Status/1(IMU1_valid), IMU_Select/5(IMU1_Valid)
  IMU_Status/1(status) -> Compare To Zero/1, IMU_status/1
  IMU2_valid/1 -> IMU_Status/2(IMU2_valid)
  IMU1_gyr_B_radPs/1 -> IMU_Select/1(IMU1_gyr_B_radPs)
  IMU2_gyr_B_radPs/1 -> IMU_Select/2(IMU2_gyr_B_radPs)
  IMU1_acc_B_mPs2/1 -> IMU_Select/3(IMU1_acc_B_mPs2)
  IMU2_acc_B_mPs2/1 -> IMU_Select/4(IMU2_acc_B_mPs2)
  IMU_Select/1(gyr_B_radPs) -> gyr_B_radPs/1
  IMU_Select/2(acc_B_mPs2) -> acc_B_mPs2/1

== system Base_INS/Sensor_Process/IMU_Process/IMU1_Scaling ==
  IMU1 : Inport  Interpolate=off  BusOutputAsStruct=on
  Acc_Calibrate : Subsystem
  Bus Selector1 : BusSelector  OutputSignals=gyr_x,gyr_y,gyr_z,acc_x,acc_y,acc_z,timestamp
  Gyro_Calibrate : Subsystem
  Vector Concatenate : Concatenate  NumInputs=3  Mode=Multidimensional array
  Vector Concatenate1 : Concatenate  NumInputs=3  Mode=Multidimensional array
  gyr_B_radDs : Outport
  acc_B_mDs2 : Outport  Port=2
  timestamp_ms : Outport  Port=3
  wires:
  Bus Selector1/1 -> Vector Concatenate/1  "<gyr_x>"
  Bus Selector1/2 -> Vector Concatenate/2  "<gyr_y>"
  Bus Selector1/3 -> Vector Concatenate/3  "<gyr_z>"
  Bus Selector1/4 -> Vector Concatenate1/1  "<acc_x>"
  Bus Selector1/5 -> Vector Concatenate1/2  "<acc_y>"
  Bus Selector1/6 -> Vector Concatenate1/3  "<acc_z>"
  Bus Selector1/7 -> timestamp_ms/1  "<timestamp>"
  IMU1/1 -> Bus Selector1/1
  Vector Concatenate/1 -> Gyro_Calibrate/1(gyro_raw)
  Vector Concatenate1/1 -> Acc_Calibrate/1(acc_raw)
  Gyro_Calibrate/1(gyr_calib) -> gyr_B_radDs/1
  Acc_Calibrate/1(acc_calib) -> acc_B_mDs2/1

== system Base_INS/Sensor_Process/IMU_Process/IMU1_Valid_Check ==
  gyr_B_radDs : Inport
  acc_B_mDs2 : Inport  Port=2
  timestamp_ms : Inport  Port=3
  Compare To Constant4 : simulink/Logic and Bit Operations/Compare To Constant  relop=<  const=timeout  OutDataTypeStr=boolean
  Constant : Constant  Value=INS_EXPORT.period  OutDataTypeStr=single
  Detect Change : simulink/Logic and Bit Operations/Detect Change  vinit=0  OutDataTypeStr=boolean
  Discrete-Time Integrator : DiscreteIntegrator  IntegratorMethod=Accumulation: Forward Euler  ExternalReset=sampled level  SampleTime=-1  OutDataTypeStr=uint32  SaturateOnIntegerOverflow=on  ICPrevOutput=DiscIntNeverNeededParam  ICPrevScaledInput=DiscIntNeverNeededParam
  Interval Test1 : simulink/Logic and Bit Operations/Interval Test  IntervalClosedRight=off  uplimit=acc_max  IntervalClosedLeft=off  lowlimit=acc_min  OutDataTypeStr=boolean
  Interval Test3 : simulink/Logic and Bit Operations/Interval Test  IntervalClosedRight=off  uplimit=gyr_max  IntervalClosedLeft=off  lowlimit=gyr_min  OutDataTypeStr=boolean
  Logical Operator : Logic  AllPortsSameDT=off  OutDataTypeStr=boolean
  Logical Operator1 : Logic  Inputs=1  AllPortsSameDT=off  OutDataTypeStr=boolean
  Logical Operator2 : Logic  Inputs=1  AllPortsSameDT=off  OutDataTypeStr=boolean
  Logical Operator4 : Logic  AllPortsSameDT=off  OutDataTypeStr=boolean
  valid : Outport
  wires:
  Logical Operator4/1 -> valid/1
  Compare To Constant4/1 -> Logical Operator4/2
  Discrete-Time Integrator/1 -> Compare To Constant4/1
  Detect Change/1 -> Discrete-Time Integrator/2
  Constant/1 -> Discrete-Time Integrator/1
  Logical Operator/1 -> Logical Operator4/1
  timestamp_ms/1 -> Detect Change/1
  Interval Test1/1 -> Logical Operator2/1
  gyr_B_radDs/1 -> Interval Test3/1
  Interval Test3/1 -> Logical Operator1/1
  Logical Operator1/1 -> Logical Operator/1
  Logical Operator2/1 -> Logical Operator/2
  acc_B_mDs2/1 -> Interval Test1/1

== system Base_INS/Sensor_Process/IMU_Process/IMU2_Scaling ==
  IMU2 : Inport  Interpolate=off  BusOutputAsStruct=on
  Acc_Calibrate : Subsystem
  Bus Selector1 : BusSelector  OutputSignals=gyr_x,gyr_y,gyr_z,acc_x,acc_y,acc_z,timestamp
  Gyro_Calibrate : Subsystem
  Vector Concatenate : Concatenate  NumInputs=3  Mode=Multidimensional array
  Vector Concatenate1 : Concatenate  NumInputs=3  Mode=Multidimensional array
  gyr_B_radDs : Outport
  acc_B_mDs2 : Outport  Port=2
  timestamp_ms : Outport  Port=3
  wires:
  Bus Selector1/1 -> Vector Concatenate/1  "<gyr_x>"
  Bus Selector1/2 -> Vector Concatenate/2  "<gyr_y>"
  Bus Selector1/3 -> Vector Concatenate/3  "<gyr_z>"
  Bus Selector1/4 -> Vector Concatenate1/1  "<acc_x>"
  Bus Selector1/5 -> Vector Concatenate1/2  "<acc_y>"
  Bus Selector1/6 -> Vector Concatenate1/3  "<acc_z>"
  Bus Selector1/7 -> timestamp_ms/1  "<timestamp>"
  IMU2/1 -> Bus Selector1/1
  Vector Concatenate/1 -> Gyro_Calibrate/1(gyro_raw)
  Vector Concatenate1/1 -> Acc_Calibrate/1(acc_raw)
  Gyro_Calibrate/1(gyr_calib) -> gyr_B_radDs/1
  Acc_Calibrate/1(acc_calib) -> acc_B_mDs2/1

== system Base_INS/Sensor_Process/IMU_Process/IMU2_Valid_Check ==
  gyr_B_radDs : Inport
  acc_B_mDs2 : Inport  Port=2
  timestamp_ms : Inport  Port=3
  Compare To Constant4 : simulink/Logic and Bit Operations/Compare To Constant  relop=<  const=timeout  OutDataTypeStr=boolean
  Constant : Constant  Value=INS_EXPORT.period  OutDataTypeStr=single
  Detect Change : simulink/Logic and Bit Operations/Detect Change  vinit=0  OutDataTypeStr=boolean
  Discrete-Time Integrator : DiscreteIntegrator  IntegratorMethod=Accumulation: Forward Euler  ExternalReset=sampled level  SampleTime=-1  OutDataTypeStr=uint32  SaturateOnIntegerOverflow=on  ICPrevOutput=DiscIntNeverNeededParam  ICPrevScaledInput=DiscIntNeverNeededParam
  Interval Test1 : simulink/Logic and Bit Operations/Interval Test  IntervalClosedRight=off  uplimit=acc_max  IntervalClosedLeft=off  lowlimit=acc_min  OutDataTypeStr=boolean
  Interval Test3 : simulink/Logic and Bit Operations/Interval Test  IntervalClosedRight=off  uplimit=gyr_max  IntervalClosedLeft=off  lowlimit=gyr_min  OutDataTypeStr=boolean
  Logical Operator : Logic  AllPortsSameDT=off  OutDataTypeStr=boolean
  Logical Operator1 : Logic  Inputs=1  AllPortsSameDT=off  OutDataTypeStr=boolean
  Logical Operator2 : Logic  Inputs=1  AllPortsSameDT=off  OutDataTypeStr=boolean
  Logical Operator4 : Logic  AllPortsSameDT=off  OutDataTypeStr=boolean
  valid : Outport
  wires:
  acc_B_mDs2/1 -> Interval Test1/1
  Logical Operator2/1 -> Logical Operator/2
  Logical Operator1/1 -> Logical Operator/1
  Interval Test3/1 -> Logical Operator1/1
  gyr_B_radDs/1 -> Interval Test3/1
  Interval Test1/1 -> Logical Operator2/1
  timestamp_ms/1 -> Detect Change/1
  Logical Operator/1 -> Logical Operator4/1
  Constant/1 -> Discrete-Time Integrator/1
  Detect Change/1 -> Discrete-Time Integrator/2
  Discrete-Time Integrator/1 -> Compare To Constant4/1
  Compare To Constant4/1 -> Logical Operator4/2
  Logical Operator4/1 -> valid/1

== system Base_INS/Sensor_Process/Mag_Process/Mag_Scaling ==
  mag_B_gauss : Inport
  Gauss_to_uT : Gain  Gain=100
  Mag_Calibrate : Subsystem
  mag_B_uT : Outport
  wires:
  Gauss_to_uT/1 -> mag_B_uT/1
  mag_B_gauss/1 -> Mag_Calibrate/1(mag_raw)
  Mag_Calibrate/1(mag_calib) -> Gauss_to_uT/1

== system Base_INS/Sensor_Process/Mag_Process/Mag_Valid_Check ==
  mag_B_gauss : Inport
  timestamp_ms : Inport  Port=2
  Compare To Constant4 : simulink/Logic and Bit Operations/Compare To Constant  relop=<  const=timeout  OutDataTypeStr=boolean
  Constant : Constant  Value=INS_EXPORT.period  OutDataTypeStr=single
  Detect Change : simulink/Logic and Bit Operations/Detect Change  vinit=0  OutDataTypeStr=boolean
  Discrete-Time Integrator : DiscreteIntegrator  IntegratorMethod=Accumulation: Forward Euler  ExternalReset=sampled level  SampleTime=-1  OutDataTypeStr=uint32  SaturateOnIntegerOverflow=on  ICPrevOutput=DiscIntNeverNeededParam  ICPrevScaledInput=DiscIntNeverNeededParam
  Interval Test1 : simulink/Logic and Bit Operations/Interval Test  IntervalClosedRight=off  uplimit=mag_max  IntervalClosedLeft=off  lowlimit=mag_min  OutDataTypeStr=boolean
  Logical Operator1 : Logic  Inputs=1  AllPortsSameDT=off  OutDataTypeStr=boolean
  Logical Operator4 : Logic  AllPortsSameDT=off  OutDataTypeStr=boolean
  valid : Outport
  wires:
  Logical Operator4/1 -> valid/1
  Compare To Constant4/1 -> Logical Operator4/2
  Discrete-Time Integrator/1 -> Compare To Constant4/1
  Detect Change/1 -> Discrete-Time Integrator/2
  Constant/1 -> Discrete-Time Integrator/1
  Logical Operator1/1 -> Logical Operator4/1
  timestamp_ms/1 -> Detect Change/1
  mag_B_gauss/1 -> Interval Test1/1
  Interval Test1/1 -> Logical Operator1/1

== system Base_INS/Sensor_Process/Mag_Process/Magnetometer ==
  mag_B_uT : Inport
  Mag_valid : Inport  Port=2
  M_OB : Inport  Port=3
  GPS_Data : Inport  Port=4
  Bus Selector : BusSelector  OutputSignals=lat_0_rad,lon_0_rad
  Bus Selector1 : BusSelector  OutputSignals=GPS_reset
  Compare To Constant : simulink/Logic and Bit Operations/Compare To Constant  relop===  const=0  OutDataTypeStr=boolean
  Quality_Indication : Subsystem
  WMM_Compensation : Subsystem
  wmm_lookup : Subsystem  mask{wmm_magnitude=INS_CONST.wmm_mag, wmm_declination=INS_CONST.wmm_dec, wmm_inclination=INS_CONST.wmm_inc, res=10}
      mask prompts: wmm_magnitude "WMM Magnitude Lookup Table"; wmm_declination "WMM Declination Lookup Table"; wmm_inclination "WMM Inclination Lookup Table"; res "Resolution"
  mag_normalized_B : Outport
  mag_Quality : Outport  Port=2
  wires:
  Quality_Indication/1(mag_quality) -> mag_Quality/1
  wmm_lookup/3(inclination_deg) -> Quality_Indication/2(nominal_Inclination_deg)
  mag_B_uT/1 -> WMM_Compensation/4(mag_B_uT)
  M_OB/1 -> WMM_Compensation/3(M_OB)
  WMM_Compensation/2(mag_normalized_O) -> Quality_Indication/1(mag_normalized_O)
  wmm_lookup/1(magnitude_uT) -> WMM_Compensation/1(magnitude_uT)
  wmm_lookup/2(declination_deg) -> WMM_Compensation/2(declination_deg)
  GPS_Data/1 -> Bus Selector1/1, Bus Selector/1
  Bus Selector/1 -> wmm_lookup/1(lat_rad)  "<lat_0_rad>"
  Bus Selector/2 -> wmm_lookup/2(lon_rad)  "<lon_0_rad>"
  Bus Selector1/1 -> Compare To Constant/1  "<GPS_reset>"
  Compare To Constant/1 -> WMM_Compensation/5(gps_available), Quality_Indication/3(gps_available)
  Mag_valid/1 -> Quality_Indication/4(mag_available)
  WMM_Compensation/1(mag_normalized_B) -> mag_normalized_B/1
